simulink model "ADRC_TD"  (R2018b)
settings: Solver=VariableStepAuto  StartTime=0.0  StopTime=100  RelTol=1e-3
settings Model: Creator=ILQMN  LastModifiedBy=ILQMN

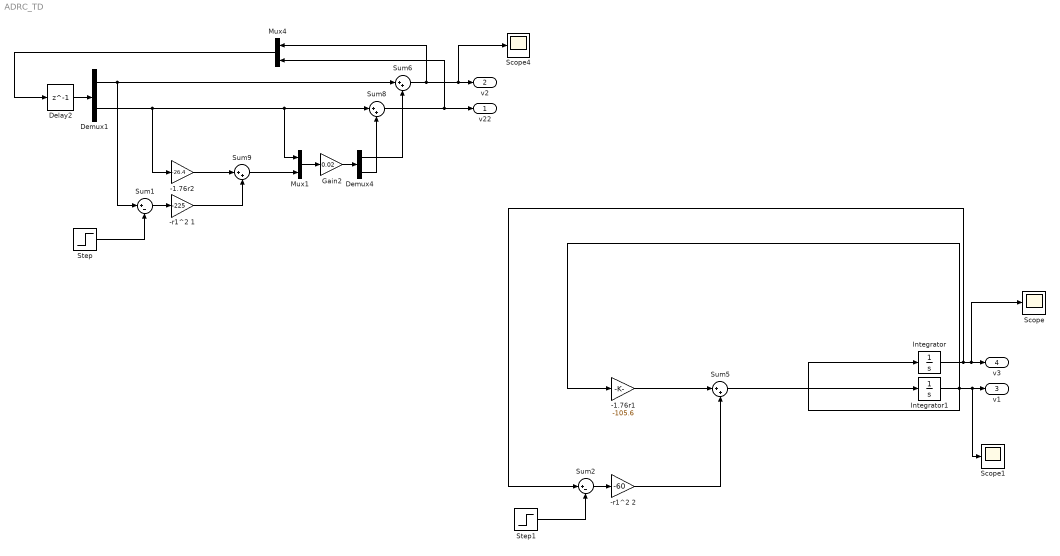
== system ADRC_TD ==
  -1.76r1 : Gain  Gain=-105.6
  -1.76r2 : Gain  Gain=-26.4
  -r1^2 1 : Gain  Gain=-225
  -r1^2 2 : Gain  Gain=-60
  Delay2 : Delay  DelayLength=1
  Demux1 : Demux  Outputs=2
  Demux4 : Demux  Outputs=2
  Gain2 : Gain  Gain=0.02
  Integrator : Integrator
  Integrator1 : Integrator
  Mux1 : Mux  Inputs=2
  Mux4 : Mux  Inputs=2
  Scope : Scope
  Scope1 : Scope
  Scope4 : Scope
  Step : Step  Time=0  SampleTime=0
  Step1 : Step  Time=0  SampleTime=0
  Sum1 : Sum  Inputs=|+-
  Sum2 : Sum  Inputs=|+-
  Sum{5..6,8..9} (4 alike) : Sum  Inputs=|++
  v22 : Outport
  v2 : Outport  Port=2
  v1 : Outport  Port=3
  v3 : Outport  Port=4
  wires:
  Demux1/1 -> Sum6/1, Sum1/1
  Mux1/1 -> Gain2/1
  Sum9/1 -> Mux1/2
  Gain2/1 -> Demux4/1
  -r1^2 1/1 -> Sum9/2
  Delay2/1 -> Demux1/1
  Sum6/1 -> Scope4/1, v2/1, Mux4/1
  Sum8/1 -> v22/1, Mux4/2
  Sum1/1 -> -r1^2 1/1
  Step/1 -> Sum1/2
  Demux4/1 -> Sum6/2
  Mux4/1 -> Delay2/1
  -1.76r2/1 -> Sum9/1
  Demux1/2 -> -1.76r2/1, Mux1/1, Sum8/1
  Demux4/2 -> Sum8/2
  -1.76r1/1 -> Sum5/1
  Sum2/1 -> -r1^2 2/1
  -r1^2 2/1 -> Sum5/2
  Step1/1 -> Sum2/2
  Integrator/1 -> Sum2/1, Scope/1, v3/1
  Integrator1/1 -> Integrator/1, Scope1/1, v1/1, -1.76r1/1
  Sum5/1 -> Integrator1/1
